simulink model "spr_od_stanu"  (R2022b)
settings: Solver=VariableStepAuto  StartTime=0.0  StopTime=1  RelTol=1e-3
values from neighbouring files (symbols this model uses):
  a21 = 1/2/m * x30^2 * FemP1/FemP2^2 * exp(-x10/FemP2)    [init.m]    (also in proj.m)
  a23 = -1/m * x30 * FemP1/FemP2 * exp(-x10/FemP2)    [init.m]    (also in proj.m)
  a31 = 1/f1 * exp(x10/f2) * (ki*u10 + ci - x30)    [init.m]    (also in proj.m)
  a33 = -f2/f1 * exp(x10/f2)    [init.m]    (also in proj.m)
  b31 = ki * f2/f1 * exp(x10/f2)    [init.m]    (also in proj.m)
  g = 9.81    [init.m]    (also in proj.m)
  K = place(A, B(:, 1), [-28, -60, -90])    [init.m]    (also in proj.m)
  u10 = 1/ki*(x30-ci)    [init.m]    (also in proj.m)
  xd = d-bd    [init.m]    (also in proj.m)
settings Model: Creator=TheZl  LastModifiedBy=pzach

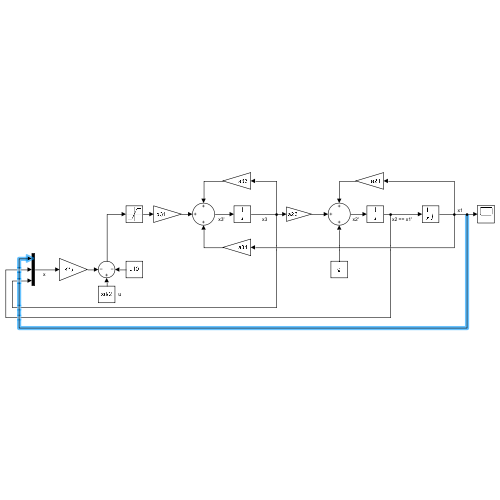
[thumbnail: Simulink's stored preview of the top-level diagram]
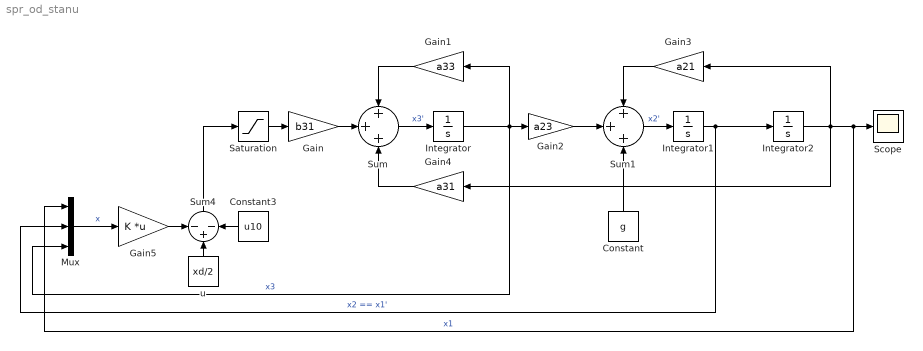
== system spr_od_stanu ==
  Constant : Constant  Value=g
  Constant3 : Constant  Value=u10
  Gain : Gain  Gain=b31
  Gain1 : Gain  Gain=a33
  Gain2 : Gain  Gain=a23
  Gain3 : Gain  Gain=a21
  Gain4 : Gain  Gain=a31
  Gain5 : Gain  Gain=K  Multiplication=Matrix(K*u)
  Integrator : Integrator
  Integrator1 : Integrator
  Integrator2 : Integrator  InitialCondition=xd  LimitOutput=on  UpperSaturationLimit=xd  LowerSaturationLimit=0
  Mux : Mux  Inputs=3
  Saturation : Saturate  UpperLimit=1  LowerLimit=0
  Scope : Scope
  Sum : Sum  Inputs=+++
  Sum1 : Sum  Inputs=+++
  Sum4 : Sum  Inputs=-+-
  u : Constant  Value=xd/2
  wires:
  Mux/1 -> Gain5/1  "x"
  u/1 -> Sum4/2
  Gain5/1 -> Sum4/1
  Constant3/1 -> Sum4/3
  Sum4/1 -> Saturation/1
  Integrator/1 -> Mux/3, Gain1/1, Gain2/1  "x3"
  Saturation/1 -> Gain/1
  Constant/1 -> Sum1/3
  Gain4/1 -> Sum/3
  Integrator1/1 -> Mux/2, Integrator2/1  "x2 == x1'"
  Sum/1 -> Integrator/1  "x3'"
  Gain1/1 -> Sum/1
  Gain3/1 -> Sum1/1
  Integrator2/1 -> Mux/1, Scope/1, Gain4/1, Gain3/1  "x1"
  Sum1/1 -> Integrator1/1  "x2'"
  Gain/1 -> Sum/2
  Gain2/1 -> Sum1/2
